simulink model "SS_MIMO_DU_Perturbacion_Simulink"  (R2019a)
settings: Solver=ode45  StartTime=0.0  StopTime=20  RelTol=1e-3
InitFcn:
  | J1=0.001;
  | B1=0.05;
  | Km1=1;
  | 
  | J2=0.002;
  | B2=0.03;
  | Km2=1;
  | Kl=10;
values from neighbouring files (symbols this model uses):
  Td = (J1/B1)/10    (= 0.002)    [IniVar.m]    (also in Initialization_MPC_SS.m = Td)
undefined symbols (not defined in the file or in its folder): nu, ny
settings Model: Creator=asierzubizarreta  LastModifiedBy=asierzubizarreta
settings DataIOCC: LimitDataPoints=on  SaveFormat=Array  ReturnWorkspaceOutputs=off
settings OptimizationCC: BlockReduction=off  BooleanDataType=off  LifeSpan=inf
settings DebuggingCC: SaveWithParameterizedLinksMsg=none  UnderspecifiedInitializationDetection=Classic  MergeDetectMultiDrivingBlocksExec=none  SignalResolutionControl=TryResolveAllWithWarning  SFUnexpectedBacktrackingDiag=warning  SFNoUnconditionalDefaultTransitionDiag=warning  SFExecutionAtInitializationDiag=none  ArithmeticOperatorsInVariantConditions=warning
settings HardwareCC: ProdBitPerPointer=32  ProdBitPerSizeT=32  ProdBitPerPtrDiffT=32  ProdLargestAtomicFloat=None  ProdIntDivRoundTo=Undefined  ProdEndianess=Unspecified  ProdWordSize=32  ProdHWDeviceType=32-bit Generic  TargetUnknown=on
settings ModelReferenceCC: PropagateSignalLabelsOutOfModel=off
settings SFSimCC: SimUseLocalCustomCode=off
settings RTWCC: RTWUseLocalCustomCode=off
settings CodeAppCC: StateflowObjectComments=on
settings GRTTargetCC: TargetLangStandard=C89/C90 (ANSI)
settings ConfigComp: CovMetricSettings=dw  CovSaveCumulativeToWorkspaceVar=on  CovSaveSingleToWorkspaceVar=on  CovExternalEMLEnable=off  CovSFcnEnable=off

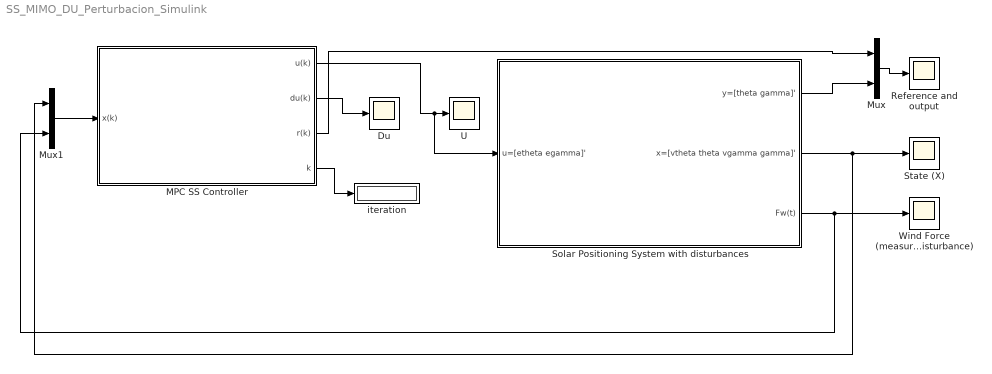
== system SS_MIMO_DU_Perturbacion_Simulink ==
  Du : Scope
  MPC SS Controller : Subsystem  InitFcn=|  TreatAsAtomicUnit=on
      | [parameters, Ref,Td]=Initialization_MPC_SS; 
      | [nx,nu]=size(parameters.B);
      | [ny,nx]=size(parameters.C);
      mask DialogControl DescGroupVar Prompt: MIMO MPC Controller
      mask DialogControl DescTextVar Prompt: This block implements a unconstrained MPC controller. du(k) is optimized
      mask Display:
      | fprintf('MPC SS Control\n\n\n');
      | 
      | 
      | port_label('output',1,'u(k)');
      | port_label('output',2,'du(k)');
      | port_label('output',3,'r(k)');
      | port_label('output',4,'k');
      | port_label('input',1,'x(k)');
  Mux : Mux  Inputs=2
  Mux1 : Mux  Inputs=2
  Reference and output : Scope
  Solar Positioning System with disturbances : Subsystem  InitFcn=|  SystemSampleTime=Td  mask{Km1=1, Jm1=0.001, B1=0.05, Km2=1, Jm2=0.002, B2=0.03, Kl=10, Kp1=0.5, Kp2=0.75, SelectorPertMeasurable=off}
      | %Inicializo random generator para el ruido
      | tcluster=clock;
      | timeseed=tcluster(6);
      mask prompts: Km1 "Motor 1 Constant (Km1)"; Jm1 "Motor 1 inertia (Jm1)"; B1 "Motor 1 Friction (B1)"; Km2 "Motor 2 Constant (Km2)"; Jm2 "Motor 2 Inertia (Jm2)"; B2 "Motor 2 Friction (B2)"; Kl "Coupling Constant (Kl)"; Kp1 "Disturbance Constant (Kp1)"; Kp2 "Disturbance Constant (Kp2)"; SelectorPertMeasurable "Measurable Disturbance ON"
      mask DialogControl Container3 Prompt: Disturbances
  State (X) : Scope
  U : Scope
  Wind Force (measurable disturbance) : Scope
  iteration : Display
  wires:
  Mux/1 -> Reference and output/1
  MPC SS Controller/4(k) -> iteration/1
  MPC SS Controller/2(du(k)) -> Du/1
  MPC SS Controller/1(u(k)) -> U/1, Solar Positioning System with disturbances/1(u=[etheta egamma]')
  Solar Positioning System with disturbances/3(Fw(t)) -> Mux1/2, Wind Force (measurable disturbance)/1
  Solar Positioning System with disturbances/1(y=[theta gamma]') -> Mux/2
  MPC SS Controller/3(r(k)) -> Mux/1
  Solar Positioning System with disturbances/2(x=[vtheta theta vgamma gamma]') -> State (X)/1, Mux1/1
  Mux1/1 -> MPC SS Controller/1(x(k))

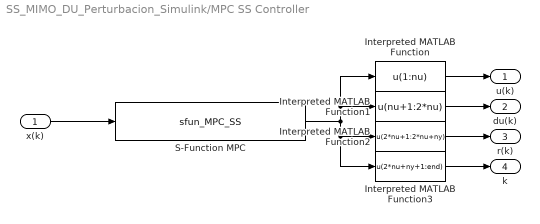
== system SS_MIMO_DU_Perturbacion_Simulink/MPC SS Controller ==
  x(k) : Inport
  Interpreted MATLAB Function : MATLABFcn  MATLABFcn=u(1:nu)
  Interpreted MATLAB Function1 : MATLABFcn  MATLABFcn=u(nu+1:2*nu)
  Interpreted MATLAB Function2 : MATLABFcn  MATLABFcn=u(2*nu+1:2*nu+ny)
  Interpreted MATLAB Function3 : MATLABFcn  MATLABFcn=u(2*nu+ny+1:end)
  S-Function MPC : S-Function  FunctionName=sfun_MPC_SS  SFunctionModules=s  SFunctionDeploymentMode=off  EnableBusSupport=off
  u(k) : Outport
  du(k) : Outport  Port=2
  r(k) : Outport  Port=3
  k : Outport  Port=4
  wires:
  Interpreted MATLAB Function/1 -> u(k)/1
  Interpreted MATLAB Function1/1 -> du(k)/1
  Interpreted MATLAB Function2/1 -> r(k)/1
  Interpreted MATLAB Function3/1 -> k/1
  x(k)/1 -> S-Function MPC/1
  S-Function MPC/1 -> Interpreted MATLAB Function1/1, Interpreted MATLAB Function/1, Interpreted MATLAB Function3/1, Interpreted MATLAB Function2/1

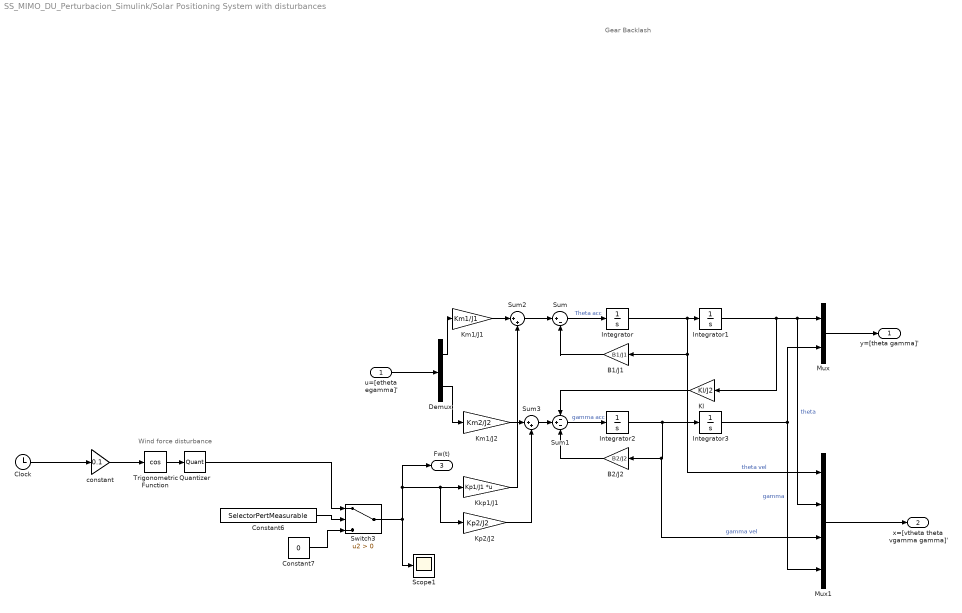
== system SS_MIMO_DU_Perturbacion_Simulink/Solar Positioning System with disturbances ==
  note: Gear Backlash
  note: Wind force disturbance
  u=[etheta egamma]' : Inport
  B1/J1 : Gain  Gain=B1/J1
  B2/J2 : Gain  Gain=B2/J2
  Clock : Clock
  Constant6 : Constant  Value=SelectorPertMeasurable
  Constant7 : Constant  Value=0
  Demux : Demux  Outputs=2
  Integrator{,1..3} (4 alike) : Integrator
  Kkp1/J1 : Gain  Gain=Kp1/J1  Multiplication=Matrix(K*u)
  Kl : Gain  Gain=Kl/J2
  Km1/J1 : Gain  Gain=Km1/J1
  Km1/J2 : Gain  Gain=Km2/J2
  Kp2/J2 : Gain  Gain=Kp2/J2
  Mux : Mux  Inputs=2
  Mux1 : Mux
  Quantizer : Quantizer
  Scope1 : Scope
  Sum : Sum  Inputs=|+-
  Sum1 : Sum  Inputs=-+-
  Sum2 : Sum  Inputs=|++
  Sum3 : Sum  Inputs=|++
  Switch3 : Switch  Criteria=u2 > Threshold
  Trigonometric Function : Trigonometry  Operator=cos
  constant : Gain  Gain=0.1
  y=[theta gamma]' : Outport
  x=[vtheta theta vgamma gamma]' : Outport  Port=2
  Fw(t) : Outport  Port=3
  wires:
  B2/J2/1 -> Sum1/3
  Kl/1 -> Sum1/1
  Integrator1/1 -> Kl/1, Mux1/2, Mux/1  "theta"
  Integrator/1 -> B1/J1/1, Mux1/1, Integrator1/1  "theta vel"
  Sum/1 -> Integrator/1  "Theta acc"
  B1/J1/1 -> Sum/2
  Integrator2/1 -> Integrator3/1, Mux1/3, B2/J2/1  "gamma vel"
  Sum1/1 -> Integrator2/1  "gamma acc"
  Mux/1 -> y=[theta gamma]'/1
  Demux/1 -> Km1/J1/1
  Demux/2 -> Km1/J2/1
  u=[etheta egamma]'/1 -> Demux/1
  Mux1/1 -> x=[vtheta theta vgamma gamma]'/1
  Switch3/1 -> Fw(t)/1, Kkp1/J1/1, Kp2/J2/1, Scope1/1
  Sum2/1 -> Sum/1
  Sum3/1 -> Sum1/2
  Km1/J2/1 -> Sum3/1
  Integrator3/1 -> Mux1/4, Mux/2  "gamma"
  Trigonometric Function/1 -> Quantizer/1
  Clock/1 -> constant/1
  constant/1 -> Trigonometric Function/1
  Constant6/1 -> Switch3/2
  Constant7/1 -> Switch3/3
  Quantizer/1 -> Switch3/1
  Km1/J1/1 -> Sum2/1
  Kkp1/J1/1 -> Sum2/2
  Kp2/J2/1 -> Sum3/2
